simulink model "nms_3Dmodel"  (Simulink 9.2)
settings: Solver=ode15s  StartTime=0.0  StopTime=30  FixedStep=1e-3  RelTol=1e-3  AbsTol=1e-4  EnableMultiTasking=on
InitFcn:
  | runScripts;
values from neighbouring files (symbols this model uses):
  ankle_height = 0.08    [nms_MechInit.m]
  c = 0.05    [nms_MechInit.m]
  c_jointstop = 0.3 / (pi/180)    (= 17.1887338539)    [nms_MechInit.m]
  CtrlPar_FP = [alpha0 alpha_cd alpha_cv]    [setCtrlPar.m]
  CtrlPar_FP_R = [R_hipR0 R_hipR_cd R_hipR_cv]    [setCtrlPar.m]
  CtrlPar_LL = l_clr    [setCtrlPar.m]
  CtrlPar_St = [StPreStim St_M1 St_M2 St_M3 St_M4 St_M5]    [setCtrlPar.m]
  CtrlPar_St_R = [R_StPreStim R_St_M1 R_St_M3 R_St_M4]    [setCtrlPar.m]
  CtrlPar_Sw = [SwPreStim SwPhasePari SwPhaseParii SwCtrlPar_H SwCtrlPar_A      SwCtrlPar_Ki SwCtrlPar_Kii SwCtrlPar_Kiii SwCtrlPar_StP]    [setCtrlPar.m]
  CtrlPar_Sw_R = [R_SwPreStim R_Sw_M6]    [setCtrlPar.m]
  CtrlPar_theta0 = parBlCtrl(1)      *1*pi/180    [setCtrlPar.m]
  CtrlPar_Tr = [Tr_St_sup Tr_Sw]    [setCtrlPar.m]
  CtrlPar_Tr_R = [R_Tr_St_sup R_Tr_Sw]    [setCtrlPar.m]
  D12_F = 0.16    [nms_MechInit.m]
  D12_S = D12_S - ankle_height/2    (= 0.46)    [nms_MechInit.m]
  D12_T = D12_T - ankle_height/2    (= 0.46)    [nms_MechInit.m]
  D12z_T = 0.1    [nms_MechInit.m]
  D13_F = 0.20    (= 0.2)    [nms_MechInit.m]
  D1G_F = 0.14    [nms_MechInit.m]
  D1G_HAT = 0.35    [nms_MechInit.m]
  D1G_S = D1G_S - ankle_height/4    (= 0.28)    [nms_MechInit.m]
  D1G_T = D1G_T - ankle_height/4    (= 0.28)    [nms_MechInit.m]
  D1Gy_F = ankle_height*D1G_F/D12_F    (= 0.07)    [nms_MechInit.m]
  d_fBall = 0.1    [nms_MechInit.m]
  d_fHeel = 0.05    [nms_MechInit.m]
  DeltaThRef = 5e-3    (= 0.005)    [nms_MechInit.m]
  eref = 0.04    [nms_MechInit.m]
  FmaxBFSH = 350    [nms_MechInit.m]
  FmaxGAS = 1500    [nms_MechInit.m]
  FmaxGLU = 1500    [nms_MechInit.m]
  FmaxHAB = 3000    [nms_MechInit.m]
  FmaxHAD = 4500    [nms_MechInit.m]
  FmaxHAM = 3000    [nms_MechInit.m]
  FmaxHFL = 2000    [nms_MechInit.m]
  FmaxRF = 1200    [nms_MechInit.m]
  FmaxSOL = 4000    [nms_MechInit.m]
  FmaxTA = 800    [nms_MechInit.m]
  FmaxVAS = 6000    [nms_MechInit.m]
  In_F = 0.005    [nms_MechInit.m]
  In_HAT = 2.5    [nms_MechInit.m]
  In_S = 0.05    [nms_MechInit.m]
  In_T = 0.15    [nms_MechInit.m]
  init_a_tgt = 70*pi/180    (= 1.2217304764)    [setInitPar.m]
  init_a_tgtR = 90*pi/180    (= 1.57079632679)    [setInitPar.m]
  Inx_F = 0.0007    [nms_MechInit.m]
  Inx_HAT = 1.0    (= 1)    [nms_MechInit.m]
  Inx_S = 0.003    [nms_MechInit.m]
  Inx_T = 0.03    [nms_MechInit.m]
  Iny_F = 0.005    [nms_MechInit.m]
  Iny_HAT = 4.0    (= 4)    [nms_MechInit.m]
  Iny_S = 0.05    [nms_MechInit.m]
  Iny_T = 0.15    [nms_MechInit.m]
  K = 5    [nms_MechInit.m]
  k_gn = k_gn/2    (= 39240)    [nms_MechInit.m]
  k_gt = k_gt/2    (= 3924)    [nms_MechInit.m]
  k_pressure = m_HAT * 9.81 / DeltaThRef    (= 104967)    [nms_MechInit.m]
  leg_l = [D12_T D12_S]    [nms_MechInit.m]
  LongDelay = 0.020/2    (= 0.01)    [nms_MechInit.m]
  LongLoopDelay = 0.030    (= 0.03)    [nms_MechInit.m]
  loptBFSH = 0.12    [nms_MechInit.m]
  loptGAS = 0.05    [nms_MechInit.m]
  loptGLU = 0.11    [nms_MechInit.m]
  loptHAB = 0.09    [nms_MechInit.m]
  loptHAD = 0.10    (= 0.1)    [nms_MechInit.m]
  loptHAM = 0.10    (= 0.1)    [nms_MechInit.m]
  loptHFL = 0.11    [nms_MechInit.m]
  loptRF = 0.08    [nms_MechInit.m]
  loptSOL = 0.04    [nms_MechInit.m]
  loptTA = 0.06    [nms_MechInit.m]
  loptVAS = 0.08    [nms_MechInit.m]
  lslackBFSH = 0.10    (= 0.1)    [nms_MechInit.m]
  lslackGAS = 0.40    (= 0.4)    [nms_MechInit.m]
  lslackGLU = 0.13    [nms_MechInit.m]
  lslackHAB = 0.07    [nms_MechInit.m]
  lslackHAD = 0.18    [nms_MechInit.m]
  lslackHAM = 0.31    [nms_MechInit.m]
  lslackHFL = 0.10    (= 0.1)    [nms_MechInit.m]
  lslackRF = 0.35    [nms_MechInit.m]
  lslackSOL = 0.26    [nms_MechInit.m]
  lslackTA = 0.24    [nms_MechInit.m]
  lslackVAS = 0.23    [nms_MechInit.m]
  m_F = 1.25    [nms_MechInit.m]
  m_HAT = 53.5    [nms_MechInit.m]
  m_S = 3.5    [nms_MechInit.m]
  m_T = 8.5    [nms_MechInit.m]
  MidDelay = 0.010/2    (= 0.005)    [nms_MechInit.m]
  mu_slide = 0.8    [nms_MechInit.m]
  mu_stick = 0.9    [nms_MechInit.m]
  N = 1.5    [nms_MechInit.m]
  phi12_LowLimit = 70*pi/180    (= 1.2217304764)    [nms_MechInit.m]
  phi12_UpLimit = 130*pi/180    (= 2.26892802759)    [nms_MechInit.m]
  phi23_UpLimit = 175*pi/180    (= 3.05432619099)    [nms_MechInit.m]
  phi34_UpLimit = 230*pi/180    (= 4.01425727959)    [nms_MechInit.m]
  phi34R_LowLimit = -15*pi/180    (= -0.261799387799)    [nms_MechInit.m]
  phi34R_UpLimit = 50*pi/180    (= 0.872664625997)    [nms_MechInit.m]
  phimaxGASa = 100*pi/180    (= 1.74532925199)    [nms_MechInit.m]
  phimaxGASk = 140*pi/180    (= 2.44346095279)    [nms_MechInit.m]
  phimaxRFk = 165*pi/180    (= 2.87979326579)    [nms_MechInit.m]
  phimaxSOL = 100*pi/180    (= 1.74532925199)    [nms_MechInit.m]
  phimaxTA = 80*pi/180    (= 1.3962634016)    [nms_MechInit.m]
  phimaxVAS = 165*pi/180    (= 2.87979326579)    [nms_MechInit.m]
  phirefBFSH = 160*pi/180    (= 2.79252680319)    [nms_MechInit.m]
  phirefGASa = 80*pi/180    (= 1.3962634016)    [nms_MechInit.m]
  phirefGASk = 165*pi/180    (= 2.87979326579)    [nms_MechInit.m]
  phirefGLU = 120*pi/180    (= 2.09439510239)    [nms_MechInit.m]
  phirefHAB = 10*pi/180    (= 0.174532925199)    [nms_MechInit.m]
  phirefHAD = 15*pi/180    (= 0.261799387799)    [nms_MechInit.m]
  phirefHAMh = 150*pi/180    (= 2.61799387799)    [nms_MechInit.m]
  phirefHAMk = 180*pi/180    (= 3.14159265359)    [nms_MechInit.m]
  phirefHFL = 160*pi/180    (= 2.79252680319)    [nms_MechInit.m]
  phirefRFh = 170*pi/180    (= 2.96705972839)    [nms_MechInit.m]
  phirefRFk = 125*pi/180    (= 2.18166156499)    [nms_MechInit.m]
  phirefSOL = 90*pi/180    (= 1.57079632679)    [nms_MechInit.m]
  phirefTA = 110*pi/180    (= 1.91986217719)    [nms_MechInit.m]
  phirefVAS = 120*pi/180    (= 2.09439510239)    [nms_MechInit.m]
  phiScaleGASa = acos(rGASamin/rGASamax)/(phiminGASa-phimaxGASa)    [nms_MechInit.m]
  phiScaleGASk = acos(rGASkmin/rGASkmax)/(phiminGASk-phimaxGASk)    [nms_MechInit.m]
  phiScaleRFk = acos(rRFkmin/rRFkmax)/(phiminRFk-phimaxRFk)    [nms_MechInit.m]
  phiScaleSOL = acos(rSOLmin/rSOLmax)/(phiminSOL-phimaxSOL)    [nms_MechInit.m]
  phiScaleTA = acos(rTAmin/rTAmax)/(phiminTA-phimaxTA)    [nms_MechInit.m]
  ... (+74 more)
undefined symbols (not defined in the file or in its folder): magnitude, sgn
libraries: mblibv1 x88, simulink x44, simulink_extras x38
(part 14 of 14)

== system nms_3Dmodel/Body Mechanics Layer/RMHeel Cnt/3D Contact/Static Friction Model ==
  note: Stiction Limit Detector
  note: Static Friction Model
  note: Zero multiplication prevents
      | horizontal friction model from
      | oscillating between static and kinetic
      | friction when the vertical force is zero but
      | the ground level is not yet reached
      | in the upward motion
  note: (distance to
      | surface)
  note: Tangential Ground Reaction Force
  pos [m] : Inport
  vel [m/s m/s m/s] : Inport  Port=2
  RefPtFP [m m m] : Inport  Port=3
  posFP [m] : Inport  Port=4
  nVecFP [m m m] : Inport  Port=5
  Enable : EnablePort  StatesWhenEnabling=reset  ZeroCross=off
  Abs : Abs
  Check Vertical Friction : Product  RndMeth=Zero
  Constant : Constant
  Dpos_n : DotProduct  InputSameDT=on  OutDataTypeStr=Inherit: Inherit via internal rule
  Dpos_nVec : Product  RndMeth=Zero
  Dpos_tVec : Sum  Inputs=|+-
  FixPt Relational Operator : RelationalOperator  Operator=>  OutDataTypeStr=boolean  ZeroCross=off  RndMeth=Nearest
  Gain : Gain  Gain=-1
  Gain1 : Gain  Gain=k_gn
  Gain2 : Gain  Gain=1/v_gn_max
  Gain3 : Gain  Gain=k_gt
  Gain5 : Gain  Gain=1/v_gt_max
  Memory : Memory
  Mux2 : Mux  Inputs=2
  Normal Ground Reaction Force : Fcn  Expr="u(1)  *  (1-u(2)) * (u(2)<1)"
  Positive : simulink/Logic and Bit Operations/Compare To Zero  relop=>  OutDataTypeStr=boolean
  Positive1 : simulink/Logic and Bit Operations/Compare To Zero  relop=>  OutDataTypeStr=boolean
  Product1 : Product  RndMeth=Zero
  Sign : Signum  ZeroCross=off
  Sum : Sum  Inputs=-+
  Sum1 : Sum  Inputs=|+-
  Sum2 : Sum  Inputs=|+-
  Vector Norm : Subsystem
  d_n : DotProduct  InputSameDT=on  OutDataTypeStr=Inherit: Inherit via internal rule
  stiction limit force : Gain  Gain=mu_stick
  sum : Sum  Inputs=++|
  tVec1 : Product  Inputs=**  RndMeth=Zero
  tVec2 : Product  Inputs=**  RndMeth=Zero
  v_n : DotProduct  InputSameDT=on  OutDataTypeStr=Inherit: Inherit via internal rule
  v_nVec : Product  RndMeth=Zero
  v_tVec : Sum  Inputs=-+|
  F_n Stick [N N N] : Outport  OutputWhenDisabled=reset  InitialOutput=[0 0 0]
      settings: AttributesFormatString=initial = '%<InitialOutput>'\nwhen disabled = '%<OutputWhenDisabled>'
  F_t Stick [N N N] : Outport  Port=2  OutputWhenDisabled=reset  InitialOutput=[0 0 0]
      settings: AttributesFormatString=when disabled: %<OutputWhenDisabled>\ninitial: %<InitialOutput>
  Sliding! : Outport  Port=3  OutputWhenDisabled=reset  InitialOutput=0
      settings: AttributesFormatString=when disabled: %<OutputWhenDisabled>\ninitial: %<InitialOutput>
  wires:
  Sum/1 -> Positive/1
  Memory/1 -> FixPt Relational Operator/2
  Positive/1 -> FixPt Relational Operator/1, Memory/1
  FixPt Relational Operator/1 -> Sliding!/1
  Abs/1 -> Sum/1
  stiction limit force/1 -> Abs/1
  Positive1/1 -> Check Vertical Friction/2
  Check Vertical Friction/1 -> Vector Norm/1(vec), F_t Stick [N N N]/1
  Normal Ground Reaction Force/1 -> Product1/2, stiction limit force/1, Positive1/1
  Mux2/1 -> Normal Ground Reaction Force/1
  Gain1/1 -> Mux2/1
  Gain2/1 -> Mux2/2
  nVecFP [m m m]/1 -> d_n/1, v_n/2, Dpos_n/1, Dpos_nVec/1, v_nVec/2, Product1/1
  d_n/1 -> Gain1/1
  vel [m/s m/s m/s]/1 -> v_tVec/2, v_n/1
  v_n/1 -> v_nVec/1, Gain2/1
  v_nVec/1 -> v_tVec/1
  v_tVec/1 -> Gain5/1
  Product1/1 -> F_n Stick [N N N]/1
  pos [m]/1 -> Sum2/1, Sum1/2
  posFP [m]/1 -> Sum2/2
  Sum2/1 -> Dpos_n/2, Dpos_tVec/1  "Dpos"
  Dpos_n/1 -> Dpos_nVec/2
  Dpos_nVec/1 -> Dpos_tVec/2
  Dpos_tVec/1 -> Gain3/1
  Gain3/1 -> Sign/1, tVec2/2
  Sign/1 -> tVec1/2
  tVec1/1 -> sum/2
  Constant/1 -> sum/1
  sum/1 -> tVec2/1
  tVec2/1 -> Gain/1
  Gain/1 -> Check Vertical Friction/1
  Vector Norm/1(norm) -> Sum/2
  RefPtFP [m m m]/1 -> Sum1/1
  Sum1/1 -> d_n/2
  Gain5/1 -> tVec1/1

== system nms_3Dmodel/Body Mechanics Layer/body pitch/roll/yaw in body frame --- x-axis: forward y-axis: leftward z-axis: parallel to gravity/new_bases/Normalize ==
  vector : Inport
  Constant1 : Constant  Value=.5
  Math Function : Math  Operator=magnitude^2  SaturateOnIntegerOverflow=on
  Product : Product  Inputs=*/  RndMeth=Zero
  Sqrt : Math  Operator=pow  OutputSignalType=real  SaturateOnIntegerOverflow=on
  Sum of Elements : Sum  Inputs=+
  unit vector : Outport
  wires:
  Sqrt/1 -> Product/2
  Sum of Elements/1 -> Sqrt/1
  Math Function/1 -> Sum of Elements/1
  vector/1 -> Product/1, Math Function/1
  Product/1 -> unit vector/1  "x_r"
  Constant1/1 -> Sqrt/2

== system nms_3Dmodel/Neural Control Layer (Spinal Cord Control)/L Swing Phase (sagittal)/kneeii_damp and hold &kneeiii_leg stop &kneeiv_stance preparation/kneeii_damp and hold ==
  note: Knee Phase i
  CtrlPar : Inport
  a_tgt : Inport  Port=2
  VceVAS : Inport  Port=3
  VceBFSH : Inport  Port=4
  VceRF : Inport  Port=5
  LceRF : Inport  Port=6
  Enable : EnablePort  StatesWhenEnabling=reset  ZeroCross=off
  Constant5 : Constant
  Demux2 : Demux  Outputs=5
  Divide1 : Product
  Divide2 : Product  Inputs=3
  Divide3 : Product  Inputs=*/
  Divide4 : Product  Inputs=*/
  Divide5 : Product
  Divide6 : Product
  Divide7 : Product  Inputs=*/
  Sum1 : Sum  Inputs=|-+  SaturateOnIntegerOverflow=on  InputSameDT=on  OutDataTypeStr=Inherit: Same as first input
  Sum10 : Sum  Inputs=|++  SaturateOnIntegerOverflow=on  InputSameDT=on  OutDataTypeStr=Inherit: Same as first input
  Sum2 : Sum  Inputs=|-+  SaturateOnIntegerOverflow=on  InputSameDT=on  OutDataTypeStr=Inherit: Same as first input
  Sum7 : Sum  Inputs=|++  SaturateOnIntegerOverflow=on  InputSameDT=on  OutDataTypeStr=Inherit: Same as first input
  positive half{,1..3} (4 alike) : Saturate  UpperLimit=inf  LowerLimit=0  ZeroCross=off
  SRF_Sw_kii : Outport  OutputWhenDisabled=reset  InitialOutput=0
  SBFSH_Sw_kii : Outport  Port=2  OutputWhenDisabled=reset  InitialOutput=0
  wires:
  CtrlPar/1 -> Demux2/1
  Demux2/1 -> Divide5/2  "VGainVAS_RF"
  VceBFSH/1 -> positive half/1, Divide3/1
  Divide5/1 -> SRF_Sw_kii/1
  positive half3/1 -> Divide5/1
  positive half/1 -> Divide1/1
  Demux2/2 -> Divide1/2  "VGainBFSH"
  Divide1/1 -> Divide2/1
  positive half1/1 -> Divide2/2
  Demux2/3 -> Divide3/2  "phi2lopt_BFSH"
  VceRF/1 -> Divide4/1
  Demux2/4 -> Divide4/2, Divide6/1, Divide7/2  "a2lopt_RF"
  Sum7/1 -> positive half1/1
  positive half2/1 -> Divide2/3
  a_tgt/1 -> Sum1/2
  Demux2/5 -> Sum1/1  "aRef_RF"
  Sum1/1 -> Divide6/2
  Divide6/1 -> Sum10/1
  Constant5/1 -> Sum10/2
  Sum10/1 -> Sum2/1  "lceOffRF"
  LceRF/1 -> Sum2/2
  Sum2/1 -> Divide7/1
  Divide7/1 -> positive half2/1
  Divide2/1 -> SBFSH_Sw_kii/1
  VceVAS/1 -> positive half3/1
  Divide3/1 -> Sum7/1
  Divide4/1 -> Sum7/2

== system nms_3Dmodel/Neural Control Layer (Spinal Cord Control)/L Swing Phase (sagittal)/kneeii_damp and hold &kneeiii_leg stop &kneeiv_stance preparation/kneeiii_leg stop ==
  note: Knee Phase iii
  CtrlPar : Inport
  a_tgt : Inport  Port=2
  LceHAM : Inport  Port=3
  Enable : EnablePort  StatesWhenEnabling=reset  ZeroCross=off
  Constant5 : Constant
  Demux1 : Demux  Outputs=7
  Divide{1..2,5,22} (4 alike) : Product
  Sum1 : Sum  Inputs=-+|  SaturateOnIntegerOverflow=on  InputSameDT=on  OutDataTypeStr=Inherit: Same as first input
  Sum10 : Sum  Inputs=+-|  SaturateOnIntegerOverflow=on  InputSameDT=on  OutDataTypeStr=Inherit: Same as first input
  Sum2 : Sum  Inputs=++|  SaturateOnIntegerOverflow=on  InputSameDT=on  OutDataTypeStr=Inherit: Same as first input
  Sum3 : Sum  Inputs=+-|  SaturateOnIntegerOverflow=on  InputSameDT=on  OutDataTypeStr=Inherit: Same as first input
  Sum4 : Sum  Inputs=+-|  SaturateOnIntegerOverflow=on  InputSameDT=on  OutDataTypeStr=Inherit: Same as first input
  positive half1 : Saturate  UpperLimit=inf  LowerLimit=0  ZeroCross=off
  positive half2 : Saturate  UpperLimit=inf  LowerLimit=0  ZeroCross=off
  SHAM_Sw_kiii : Outport  OutputWhenDisabled=reset  InitialOutput=0
  SKFL_Sw_kiii : Outport  Port=2  OutputWhenDisabled=reset  InitialOutput=0
  SGAS_Sw_kiii : Outport  Port=3  OutputWhenDisabled=reset  InitialOutput=0
  wires:
  CtrlPar/1 -> Demux1/1
  Sum1/1 -> positive half2/1  "del_LceMAN"
  LceHAM/1 -> Sum1/2  "LceHAM"
  positive half2/1 -> Divide5/1  "del_lce"
  Constant5/1 -> Sum10/1
  Divide22/1 -> Sum10/2
  a_tgt/1 -> Sum2/1
  Demux1/1 -> Sum2/2  "a_del"
  Sum2/1 -> Sum3/1  "a_thr"
  Demux1/2 -> Sum3/2  "aRef_HAM"
  Sum3/1 -> Divide22/1
  Demux1/3 -> Divide22/2  "a2lopt_HAM"
  Sum10/1 -> Sum1/1  "lceOffHAM"
  Demux1/4 -> Divide5/2  "LGainHAM"
  Divide5/1 -> Sum4/1, SHAM_Sw_kiii/1  "S_HAM"
  Sum4/1 -> positive half1/1
  Demux1/5 -> Sum4/2  "SHAM_thr"
  positive half1/1 -> Divide1/1, Divide2/1
  Demux1/6 -> Divide1/2  "SGainHAM_KFL"
  Divide1/1 -> SKFL_Sw_kiii/1
  Divide2/1 -> SGAS_Sw_kiii/1
  Demux1/7 -> Divide2/2  "SGainHAM_GAS"

== system nms_3Dmodel/Neural Control Layer (Spinal Cord Control)/L Swing Phase (sagittal)/kneeii_damp and hold &kneeiii_leg stop &kneeiv_stance preparation/kneeiv_stance preparation ==
  note: Knee Phase iii
  CtrlPar : Inport
  a_tgt : Inport  Port=2
  LceHFL : Inport  Port=3
  lceGLU : Inport  Port=4
  lceVAS : Inport  Port=5
  Enable : EnablePort  StatesWhenEnabling=reset  ZeroCross=off
  Constant1 : Constant
  Constant2 : Constant
  Constant5 : Constant  Value=pi/2
  Demux2 : Demux  Outputs=8
  Divide{1..3,5..6} (5 alike) : Product
  Sum1 : Sum  Inputs=-+|  SaturateOnIntegerOverflow=on  InputSameDT=on  OutDataTypeStr=Inherit: Same as first input
  Sum2 : Sum  Inputs=++|  SaturateOnIntegerOverflow=on  InputSameDT=on  OutDataTypeStr=Inherit: Same as first input
  Sum3 : Sum  Inputs=+-|  SaturateOnIntegerOverflow=on  InputSameDT=on  OutDataTypeStr=Inherit: Same as first input
  Sum4 : Sum  Inputs=+-|  SaturateOnIntegerOverflow=on  InputSameDT=on  OutDataTypeStr=Inherit: Same as first input
  Sum5 : Sum  Inputs=++|  SaturateOnIntegerOverflow=on  InputSameDT=on  OutDataTypeStr=Inherit: Same as first input
  Sum6 : Sum  Inputs=-+|  SaturateOnIntegerOverflow=on  InputSameDT=on  OutDataTypeStr=Inherit: Same as first input
  Sum7 : Sum  Inputs=+-|  SaturateOnIntegerOverflow=on  InputSameDT=on  OutDataTypeStr=Inherit: Same as first input
  Sum9 : Sum  Inputs=-+|  SaturateOnIntegerOverflow=on  InputSameDT=on  OutDataTypeStr=Inherit: Same as first input
  positive half1 : Saturate  UpperLimit=inf  LowerLimit=0  ZeroCross=off
  positive half2 : Saturate  UpperLimit=inf  LowerLimit=0  ZeroCross=off
  positive half3 : Saturate  UpperLimit=inf  LowerLimit=0  ZeroCross=off
  SHFL_Sw_kiv : Outport  OutputWhenDisabled=reset  InitialOutput=0
  SGLU_Sw_kiv : Outport  Port=2  OutputWhenDisabled=reset  InitialOutput=0
  SVAS_Sw_kiv : Outport  Port=3  OutputWhenDisabled=reset  InitialOutput=0
  wires:
  CtrlPar/1 -> Demux2/1
  Sum1/1 -> positive half2/1
  LceHFL/1 -> Sum1/2
  positive half2/1 -> Divide5/1
  a_tgt/1 -> Sum2/2
  Constant5/1 -> Sum2/1
  Demux2/1 -> Sum3/2  "phiRef_HFL"
  Sum2/1 -> Sum3/1, Sum4/1
  Sum3/1 -> Divide1/1
  Demux2/2 -> Divide1/2  "phi2lopt_HFL"
  Demux2/5 -> Divide2/2  "phi2lopt_GLU"
  Demux2/4 -> Sum4/2  "phiRef_GLU"
  Sum4/1 -> Divide2/1
  Demux2/3 -> Divide5/2  "LGainHFL"
  Divide5/1 -> SHFL_Sw_kiv/1
  Constant1/1 -> Sum5/1
  Divide1/1 -> Sum5/2
  Sum5/1 -> Sum1/1  "lceOffHFL"
  Sum6/1 -> positive half1/1  "del_lce"
  lceGLU/1 -> Sum6/2  "lceGLU"
  positive half1/1 -> Divide3/1
  Demux2/6 -> Divide3/2  "LGainGLU"
  Divide3/1 -> SGLU_Sw_kiv/1
  Constant2/1 -> Sum7/1
  Divide2/1 -> Sum7/2
  Sum7/1 -> Sum6/1  "lceOffGLU"
  Sum9/1 -> positive half3/1
  lceVAS/1 -> Sum9/2
  positive half3/1 -> Divide6/1
  Divide6/1 -> SVAS_Sw_kiv/1
  Demux2/7 -> Sum9/1  "loffVAS"
  Demux2/8 -> Divide6/2  "LGainVAS"

== system nms_3Dmodel/Neural Control Layer (Spinal Cord Control)/R Swing Phase (sagittal)/kneeii_damp and hold &kneeiii_leg stop &kneeiv_stance preparation/kneeii_damp and hold ==
  note: Knee Phase i
  CtrlPar : Inport
  a_tgt : Inport  Port=2
  VceVAS : Inport  Port=3
  VceBFSH : Inport  Port=4
  VceRF : Inport  Port=5
  LceRF : Inport  Port=6
  Enable : EnablePort  StatesWhenEnabling=reset  ZeroCross=off
  Constant5 : Constant
  Demux2 : Demux  Outputs=5
  Divide1 : Product
  Divide2 : Product  Inputs=3
  Divide3 : Product  Inputs=*/
  Divide4 : Product  Inputs=*/
  Divide5 : Product
  Divide6 : Product
  Divide7 : Product  Inputs=*/
  Sum1 : Sum  Inputs=|-+  SaturateOnIntegerOverflow=on  InputSameDT=on  OutDataTypeStr=Inherit: Same as first input
  Sum10 : Sum  Inputs=|++  SaturateOnIntegerOverflow=on  InputSameDT=on  OutDataTypeStr=Inherit: Same as first input
  Sum2 : Sum  Inputs=|-+  SaturateOnIntegerOverflow=on  InputSameDT=on  OutDataTypeStr=Inherit: Same as first input
  Sum7 : Sum  Inputs=|++  SaturateOnIntegerOverflow=on  InputSameDT=on  OutDataTypeStr=Inherit: Same as first input
  positive half{,1..3} (4 alike) : Saturate  UpperLimit=inf  LowerLimit=0  ZeroCross=off
  SRF_Sw_kii : Outport  OutputWhenDisabled=reset  InitialOutput=0
  SBFSH_Sw_kii : Outport  Port=2  OutputWhenDisabled=reset  InitialOutput=0
  wires:
  CtrlPar/1 -> Demux2/1
  Demux2/1 -> Divide5/2  "VGainVAS_RF"
  VceBFSH/1 -> positive half/1, Divide3/1
  Divide5/1 -> SRF_Sw_kii/1
  positive half3/1 -> Divide5/1
  positive half/1 -> Divide1/1
  Demux2/2 -> Divide1/2  "VGainBFSH"
  Divide1/1 -> Divide2/1
  positive half1/1 -> Divide2/2
  Demux2/3 -> Divide3/2  "phi2lopt_BFSH"
  VceRF/1 -> Divide4/1
  Demux2/4 -> Divide4/2, Divide6/1, Divide7/2  "a2lopt_RF"
  Sum7/1 -> positive half1/1
  positive half2/1 -> Divide2/3
  a_tgt/1 -> Sum1/2
  Demux2/5 -> Sum1/1  "aRef_RF"
  Sum1/1 -> Divide6/2
  Divide6/1 -> Sum10/1
  Constant5/1 -> Sum10/2
  Sum10/1 -> Sum2/1  "lceOffRF"
  LceRF/1 -> Sum2/2
  Sum2/1 -> Divide7/1
  Divide7/1 -> positive half2/1
  Divide2/1 -> SBFSH_Sw_kii/1
  VceVAS/1 -> positive half3/1
  Divide3/1 -> Sum7/1
  Divide4/1 -> Sum7/2

== system nms_3Dmodel/Neural Control Layer (Spinal Cord Control)/R Swing Phase (sagittal)/kneeii_damp and hold &kneeiii_leg stop &kneeiv_stance preparation/kneeiii_leg stop ==
  note: Knee Phase iii
  CtrlPar : Inport
  a_tgt : Inport  Port=2
  LceHAM : Inport  Port=3
  Enable : EnablePort  StatesWhenEnabling=reset  ZeroCross=off
  Constant5 : Constant
  Demux1 : Demux  Outputs=7
  Divide{1..2,5,22} (4 alike) : Product
  Sum1 : Sum  Inputs=-+|  SaturateOnIntegerOverflow=on  InputSameDT=on  OutDataTypeStr=Inherit: Same as first input
  Sum10 : Sum  Inputs=+-|  SaturateOnIntegerOverflow=on  InputSameDT=on  OutDataTypeStr=Inherit: Same as first input
  Sum2 : Sum  Inputs=++|  SaturateOnIntegerOverflow=on  InputSameDT=on  OutDataTypeStr=Inherit: Same as first input
  Sum3 : Sum  Inputs=+-|  SaturateOnIntegerOverflow=on  InputSameDT=on  OutDataTypeStr=Inherit: Same as first input
  Sum4 : Sum  Inputs=+-|  SaturateOnIntegerOverflow=on  InputSameDT=on  OutDataTypeStr=Inherit: Same as first input
  positive half1 : Saturate  UpperLimit=inf  LowerLimit=0  ZeroCross=off
  positive half2 : Saturate  UpperLimit=inf  LowerLimit=0  ZeroCross=off
  SHAM_Sw_kiii : Outport  OutputWhenDisabled=reset  InitialOutput=0
  SKFL_Sw_kiii : Outport  Port=2  OutputWhenDisabled=reset  InitialOutput=0
  SGAS_Sw_kiii : Outport  Port=3  OutputWhenDisabled=reset  InitialOutput=0
  wires:
  CtrlPar/1 -> Demux1/1
  Sum1/1 -> positive half2/1  "del_LceMAN"
  LceHAM/1 -> Sum1/2  "LceHAM"
  positive half2/1 -> Divide5/1  "del_lce"
  Constant5/1 -> Sum10/1
  Divide22/1 -> Sum10/2
  a_tgt/1 -> Sum2/1
  Demux1/1 -> Sum2/2  "a_del"
  Sum2/1 -> Sum3/1  "a_thr"
  Demux1/2 -> Sum3/2  "aRef_HAM"
  Sum3/1 -> Divide22/1
  Demux1/3 -> Divide22/2  "a2lopt_HAM"
  Sum10/1 -> Sum1/1  "lceOffHAM"
  Demux1/4 -> Divide5/2  "LGainHAM"
  Divide5/1 -> Sum4/1, SHAM_Sw_kiii/1  "S_HAM"
  Sum4/1 -> positive half1/1
  Demux1/5 -> Sum4/2  "SHAM_thr"
  positive half1/1 -> Divide1/1, Divide2/1
  Demux1/6 -> Divide1/2  "SGainHAM_KFL"
  Divide1/1 -> SKFL_Sw_kiii/1
  Divide2/1 -> SGAS_Sw_kiii/1
  Demux1/7 -> Divide2/2  "SGainHAM_GAS"

== system nms_3Dmodel/Neural Control Layer (Spinal Cord Control)/R Swing Phase (sagittal)/kneeii_damp and hold &kneeiii_leg stop &kneeiv_stance preparation/kneeiv_stance preparation ==
  note: Knee Phase iii
  CtrlPar : Inport
  a_tgt : Inport  Port=2
  LceHFL : Inport  Port=3
  lceGLU : Inport  Port=4
  lceVAS : Inport  Port=5
  Enable : EnablePort  StatesWhenEnabling=reset  ZeroCross=off
  Constant1 : Constant
  Constant2 : Constant
  Constant5 : Constant  Value=pi/2
  Demux2 : Demux  Outputs=8
  Divide{1..3,5..6} (5 alike) : Product
  Sum1 : Sum  Inputs=-+|  SaturateOnIntegerOverflow=on  InputSameDT=on  OutDataTypeStr=Inherit: Same as first input
  Sum2 : Sum  Inputs=++|  SaturateOnIntegerOverflow=on  InputSameDT=on  OutDataTypeStr=Inherit: Same as first input
  Sum3 : Sum  Inputs=+-|  SaturateOnIntegerOverflow=on  InputSameDT=on  OutDataTypeStr=Inherit: Same as first input
  Sum4 : Sum  Inputs=+-|  SaturateOnIntegerOverflow=on  InputSameDT=on  OutDataTypeStr=Inherit: Same as first input
  Sum5 : Sum  Inputs=++|  SaturateOnIntegerOverflow=on  InputSameDT=on  OutDataTypeStr=Inherit: Same as first input
  Sum6 : Sum  Inputs=-+|  SaturateOnIntegerOverflow=on  InputSameDT=on  OutDataTypeStr=Inherit: Same as first input
  Sum7 : Sum  Inputs=+-|  SaturateOnIntegerOverflow=on  InputSameDT=on  OutDataTypeStr=Inherit: Same as first input
  Sum9 : Sum  Inputs=-+|  SaturateOnIntegerOverflow=on  InputSameDT=on  OutDataTypeStr=Inherit: Same as first input
  positive half1 : Saturate  UpperLimit=inf  LowerLimit=0  ZeroCross=off
  positive half2 : Saturate  UpperLimit=inf  LowerLimit=0  ZeroCross=off
  positive half3 : Saturate  UpperLimit=inf  LowerLimit=0  ZeroCross=off
  SHFL_Sw_kiv : Outport  OutputWhenDisabled=reset  InitialOutput=0
  SGLU_Sw_kiv : Outport  Port=2  OutputWhenDisabled=reset  InitialOutput=0
  SVAS_Sw_kiv : Outport  Port=3  OutputWhenDisabled=reset  InitialOutput=0
  wires:
  CtrlPar/1 -> Demux2/1
  Sum1/1 -> positive half2/1
  LceHFL/1 -> Sum1/2
  positive half2/1 -> Divide5/1
  a_tgt/1 -> Sum2/2
  Constant5/1 -> Sum2/1
  Demux2/1 -> Sum3/2  "phiRef_HFL"
  Sum2/1 -> Sum3/1, Sum4/1
  Sum3/1 -> Divide1/1
  Demux2/2 -> Divide1/2  "phi2lopt_HFL"
  Demux2/5 -> Divide2/2  "phi2lopt_GLU"
  Demux2/4 -> Sum4/2  "phiRef_GLU"
  Sum4/1 -> Divide2/1
  Demux2/3 -> Divide5/2  "LGainHFL"
  Divide5/1 -> SHFL_Sw_kiv/1
  Constant1/1 -> Sum5/1
  Divide1/1 -> Sum5/2
  Sum5/1 -> Sum1/1  "lceOffHFL"
  Sum6/1 -> positive half1/1  "del_lce"
  lceGLU/1 -> Sum6/2  "lceGLU"
  positive half1/1 -> Divide3/1
  Demux2/6 -> Divide3/2  "LGainGLU"
  Divide3/1 -> SGLU_Sw_kiv/1
  Constant2/1 -> Sum7/1
  Divide2/1 -> Sum7/2
  Sum7/1 -> Sum6/1  "lceOffGLU"
  Sum9/1 -> positive half3/1
  lceVAS/1 -> Sum9/2
  positive half3/1 -> Divide6/1
  Divide6/1 -> SVAS_Sw_kiv/1
  Demux2/7 -> Sum9/1  "loffVAS"
  Demux2/8 -> Divide6/2  "LGainVAS"

== system nms_3Dmodel/Body Mechanics Layer/LLBall Cnt/3D Contact/Kinetic Friction Model/Vector Norm ==
  vec : Inport
  Constant1 : Constant  Value=.5
  Sqrt : Math  Operator=pow  OutputSignalType=real  SaturateOnIntegerOverflow=on
  Squares : Math  Operator=square  OutputSignalType=real  SaturateOnIntegerOverflow=on
  Sum of Elements : Sum  Inputs=+
  norm : Outport
  wires:
  vec/1 -> Squares/1
  Sqrt/1 -> norm/1
  Sum of Elements/1 -> Sqrt/1
  Squares/1 -> Sum of Elements/1
  Constant1/1 -> Sqrt/2

== system nms_3Dmodel/Body Mechanics Layer/LLBall Cnt/3D Contact/Static Friction Model/Vector Norm ==
  vec : Inport
  Constant1 : Constant  Value=.5
  Sqrt : Math  Operator=pow  OutputSignalType=real  SaturateOnIntegerOverflow=on
  Squares : Math  Operator=square  OutputSignalType=real  SaturateOnIntegerOverflow=on
  Sum of Elements : Sum  Inputs=+
  norm : Outport
  wires:
  vec/1 -> Squares/1
  Sqrt/1 -> norm/1
  Sum of Elements/1 -> Sqrt/1
  Squares/1 -> Sum of Elements/1
  Constant1/1 -> Sqrt/2

== system nms_3Dmodel/Body Mechanics Layer/LLHeel Cnt/3D Contact/Kinetic Friction Model/Vector Norm ==
  vec : Inport
  Constant1 : Constant  Value=.5
  Sqrt : Math  Operator=pow  OutputSignalType=real  SaturateOnIntegerOverflow=on
  Squares : Math  Operator=square  OutputSignalType=real  SaturateOnIntegerOverflow=on
  Sum of Elements : Sum  Inputs=+
  norm : Outport
  wires:
  vec/1 -> Squares/1
  Sqrt/1 -> norm/1
  Sum of Elements/1 -> Sqrt/1
  Squares/1 -> Sum of Elements/1
  Constant1/1 -> Sqrt/2

== system nms_3Dmodel/Body Mechanics Layer/LLHeel Cnt/3D Contact/Static Friction Model/Vector Norm ==
  vec : Inport
  Constant1 : Constant  Value=.5
  Sqrt : Math  Operator=pow  OutputSignalType=real  SaturateOnIntegerOverflow=on
  Squares : Math  Operator=square  OutputSignalType=real  SaturateOnIntegerOverflow=on
  Sum of Elements : Sum  Inputs=+
  norm : Outport
  wires:
  vec/1 -> Squares/1
  Sqrt/1 -> norm/1
  Sum of Elements/1 -> Sqrt/1
  Squares/1 -> Sum of Elements/1
  Constant1/1 -> Sqrt/2

== system nms_3Dmodel/Body Mechanics Layer/LMBall Cnt/3D Contact/Kinetic Friction Model/Vector Norm ==
  vec : Inport
  Constant1 : Constant  Value=.5
  Sqrt : Math  Operator=pow  OutputSignalType=real  SaturateOnIntegerOverflow=on
  Squares : Math  Operator=square  OutputSignalType=real  SaturateOnIntegerOverflow=on
  Sum of Elements : Sum  Inputs=+
  norm : Outport
  wires:
  vec/1 -> Squares/1
  Sqrt/1 -> norm/1
  Sum of Elements/1 -> Sqrt/1
  Squares/1 -> Sum of Elements/1
  Constant1/1 -> Sqrt/2

== system nms_3Dmodel/Body Mechanics Layer/LMBall Cnt/3D Contact/Static Friction Model/Vector Norm ==
  vec : Inport
  Constant1 : Constant  Value=.5
  Sqrt : Math  Operator=pow  OutputSignalType=real  SaturateOnIntegerOverflow=on
  Squares : Math  Operator=square  OutputSignalType=real  SaturateOnIntegerOverflow=on
  Sum of Elements : Sum  Inputs=+
  norm : Outport
  wires:
  vec/1 -> Squares/1
  Sqrt/1 -> norm/1
  Sum of Elements/1 -> Sqrt/1
  Squares/1 -> Sum of Elements/1
  Constant1/1 -> Sqrt/2

== system nms_3Dmodel/Body Mechanics Layer/LMHeel Cnt/3D Contact/Kinetic Friction Model/Vector Norm ==
  vec : Inport
  Constant1 : Constant  Value=.5
  Sqrt : Math  Operator=pow  OutputSignalType=real  SaturateOnIntegerOverflow=on
  Squares : Math  Operator=square  OutputSignalType=real  SaturateOnIntegerOverflow=on
  Sum of Elements : Sum  Inputs=+
  norm : Outport
  wires:
  vec/1 -> Squares/1
  Sqrt/1 -> norm/1
  Sum of Elements/1 -> Sqrt/1
  Squares/1 -> Sum of Elements/1
  Constant1/1 -> Sqrt/2

== system nms_3Dmodel/Body Mechanics Layer/LMHeel Cnt/3D Contact/Static Friction Model/Vector Norm ==
  vec : Inport
  Constant1 : Constant  Value=.5
  Sqrt : Math  Operator=pow  OutputSignalType=real  SaturateOnIntegerOverflow=on
  Squares : Math  Operator=square  OutputSignalType=real  SaturateOnIntegerOverflow=on
  Sum of Elements : Sum  Inputs=+
  norm : Outport
  wires:
  vec/1 -> Squares/1
  Sqrt/1 -> norm/1
  Sum of Elements/1 -> Sqrt/1
  Squares/1 -> Sum of Elements/1
  Constant1/1 -> Sqrt/2

== system nms_3Dmodel/Body Mechanics Layer/RLBall Cnt/3D Contact/Kinetic Friction Model/Vector Norm ==
  vec : Inport
  Constant1 : Constant  Value=.5
  Sqrt : Math  Operator=pow  OutputSignalType=real  SaturateOnIntegerOverflow=on
  Squares : Math  Operator=square  OutputSignalType=real  SaturateOnIntegerOverflow=on
  Sum of Elements : Sum  Inputs=+
  norm : Outport
  wires:
  vec/1 -> Squares/1
  Sqrt/1 -> norm/1
  Sum of Elements/1 -> Sqrt/1
  Squares/1 -> Sum of Elements/1
  Constant1/1 -> Sqrt/2

== system nms_3Dmodel/Body Mechanics Layer/RLBall Cnt/3D Contact/Static Friction Model/Vector Norm ==
  vec : Inport
  Constant1 : Constant  Value=.5
  Sqrt : Math  Operator=pow  OutputSignalType=real  SaturateOnIntegerOverflow=on
  Squares : Math  Operator=square  OutputSignalType=real  SaturateOnIntegerOverflow=on
  Sum of Elements : Sum  Inputs=+
  norm : Outport
  wires:
  vec/1 -> Squares/1
  Sqrt/1 -> norm/1
  Sum of Elements/1 -> Sqrt/1
  Squares/1 -> Sum of Elements/1
  Constant1/1 -> Sqrt/2

== system nms_3Dmodel/Body Mechanics Layer/RLHeel Cnt/3D Contact/Kinetic Friction Model/Vector Norm ==
  vec : Inport
  Constant1 : Constant  Value=.5
  Sqrt : Math  Operator=pow  OutputSignalType=real  SaturateOnIntegerOverflow=on
  Squares : Math  Operator=square  OutputSignalType=real  SaturateOnIntegerOverflow=on
  Sum of Elements : Sum  Inputs=+
  norm : Outport
  wires:
  vec/1 -> Squares/1
  Sqrt/1 -> norm/1
  Sum of Elements/1 -> Sqrt/1
  Squares/1 -> Sum of Elements/1
  Constant1/1 -> Sqrt/2

== system nms_3Dmodel/Body Mechanics Layer/RLHeel Cnt/3D Contact/Static Friction Model/Vector Norm ==
  vec : Inport
  Constant1 : Constant  Value=.5
  Sqrt : Math  Operator=pow  OutputSignalType=real  SaturateOnIntegerOverflow=on
  Squares : Math  Operator=square  OutputSignalType=real  SaturateOnIntegerOverflow=on
  Sum of Elements : Sum  Inputs=+
  norm : Outport
  wires:
  vec/1 -> Squares/1
  Sqrt/1 -> norm/1
  Sum of Elements/1 -> Sqrt/1
  Squares/1 -> Sum of Elements/1
  Constant1/1 -> Sqrt/2

== system nms_3Dmodel/Body Mechanics Layer/RMBall Cnt/3D Contact/Kinetic Friction Model/Vector Norm ==
  vec : Inport
  Constant1 : Constant  Value=.5
  Sqrt : Math  Operator=pow  OutputSignalType=real  SaturateOnIntegerOverflow=on
  Squares : Math  Operator=square  OutputSignalType=real  SaturateOnIntegerOverflow=on
  Sum of Elements : Sum  Inputs=+
  norm : Outport
  wires:
  vec/1 -> Squares/1
  Sqrt/1 -> norm/1
  Sum of Elements/1 -> Sqrt/1
  Squares/1 -> Sum of Elements/1
  Constant1/1 -> Sqrt/2

== system nms_3Dmodel/Body Mechanics Layer/RMBall Cnt/3D Contact/Static Friction Model/Vector Norm ==
  vec : Inport
  Constant1 : Constant  Value=.5
  Sqrt : Math  Operator=pow  OutputSignalType=real  SaturateOnIntegerOverflow=on
  Squares : Math  Operator=square  OutputSignalType=real  SaturateOnIntegerOverflow=on
  Sum of Elements : Sum  Inputs=+
  norm : Outport
  wires:
  vec/1 -> Squares/1
  Sqrt/1 -> norm/1
  Sum of Elements/1 -> Sqrt/1
  Squares/1 -> Sum of Elements/1
  Constant1/1 -> Sqrt/2

== system nms_3Dmodel/Body Mechanics Layer/RMHeel Cnt/3D Contact/Kinetic Friction Model/Vector Norm ==
  vec : Inport
  Constant1 : Constant  Value=.5
  Sqrt : Math  Operator=pow  OutputSignalType=real  SaturateOnIntegerOverflow=on
  Squares : Math  Operator=square  OutputSignalType=real  SaturateOnIntegerOverflow=on
  Sum of Elements : Sum  Inputs=+
  norm : Outport
  wires:
  vec/1 -> Squares/1
  Sqrt/1 -> norm/1
  Sum of Elements/1 -> Sqrt/1
  Squares/1 -> Sum of Elements/1
  Constant1/1 -> Sqrt/2

== system nms_3Dmodel/Body Mechanics Layer/RMHeel Cnt/3D Contact/Static Friction Model/Vector Norm ==
  vec : Inport
  Constant1 : Constant  Value=.5
  Sqrt : Math  Operator=pow  OutputSignalType=real  SaturateOnIntegerOverflow=on
  Squares : Math  Operator=square  OutputSignalType=real  SaturateOnIntegerOverflow=on
  Sum of Elements : Sum  Inputs=+
  norm : Outport
  wires:
  vec/1 -> Squares/1
  Sqrt/1 -> norm/1
  Sum of Elements/1 -> Sqrt/1
  Squares/1 -> Sum of Elements/1
  Constant1/1 -> Sqrt/2
